simulink model "mCounterWithReset"  (R2021b)
settings: Solver=FixedStepDiscrete  StartTime=0.0  StopTime=10.0  RelTol=1e-3
PreLoadFcn:
  | A=1;
  | 
  | % -------------------------------------------------------------------
  | %  Generated by MATLAB on 17-Oct-2019 16:20:17
  | %  MATLAB version: 9.8.0.1209737 (R2020a) Prerelease
  | % -------------------------------------------------------------------
  | 
  | 
  | main_bus = Simulink.Bus;
  | main_bus.Description = '';
  | main_bus.DataScope = 'Auto';
  | main_bus.HeaderFile = '';
  | main_bus.Alignment = -1;
  | saveVarsTmp{1} = Simulink.BusElement;
  | saveVarsTmp{1}.Name = 'Counter';
  | saveVarsTmp{1}.Complexity = 'real';
  | saveVarsTmp{1}.Dimensions = 1;
  | saveVarsTmp{1}.DataType = 'double';
  | saveVarsTmp{1}.Min = [];
  | saveVarsTmp{1}.Max = [];
  | saveVarsTmp{1}.DimensionsMode = 'Fixed';
  | saveVarsTmp{1}.SamplingMode = 'Sample based';
  | saveVarsTmp{1}.SampleTime = -1;
  | saveVarsTmp{1}.DocUnits = '';
  | saveVarsTmp{1}.Description = '';
  | saveVarsTmp{1}(2, 1) = Simulink.BusElement;
  | saveVarsTmp{1}(2, 1).Name = 'Reset';
  | saveVarsTmp{1}(2, 1).Complexity = 'real';
  | saveVarsTmp{1}(2, 1).Dimensions = 1;
  | saveVarsTmp{1}(2, 1).DataType = 'boolean';
  | saveVarsTmp{1}(2, 1).Min = [];
  | saveVarsTmp{1}(2, 1).Max = [];
  | saveVarsTmp{1}(2, 1).DimensionsMode = 'Fixed';
  | saveVarsTmp{1}(2, 1).SamplingMode = 'Sample based';
  | saveVarsTmp{1}(2, 1).SampleTime = -1;
  | saveVarsTmp{1}(2, 1).DocUnits = '';
  | saveVarsTmp{1}(2, 1).Description = '';
  | main_bus.Elements = saveVarsTmp{1};
  | clear saveVarsTmp;
CloseFcn:
  | clear A main_bus;
settings Model: Creator=nrangava  LastModifiedBy=nrangava
settings SolverCC: AlgebraicLoopSolver=TrustRegion  MaxZcPerStep=1
settings DataIOCC: SaveFormat=StructureWithTime  SaveState=on  DSMLogging=off  OutputSaveName=yout1
settings OptimizationCC: DefaultParameterBehavior=Inlined  EnhancedBackFolding=on  PassReuseOutputArgsAs=Individual arguments  ZeroExternalMemoryAtStartup=off  ZeroInternalMemoryAtStartup=off  OptimizeBlockOrder=speed  DifferentSizesBufferReuse=on  OptimizationCustomize=off  EfficientTunableParamExpr=on
settings DebuggingCC: ParameterTunabilityLossMsg=error  SFMachineParentedDataDiag=warning
settings HardwareCC: TargetBitPerPointer=64  TargetBitPerSizeT=64  TargetBitPerPtrDiffT=64  TargetLongLongMode=on  TargetIntDivRoundTo=Zero  TargetEndianess=LittleEndian  TargetWordSize=64  TargetHWDeviceType=Custom Processor->MATLAB Host Computer  ProdEqTarget=off
settings ModelReferenceCC: UpdateModelReferenceTargets=IfOutOfDate
settings SFSimCC: MATLABDynamicMemAlloc=off
settings RTWCC: Description=Embedded Coder  SystemTargetFile=ert.tlc  TemplateMakefile=ert_default_tmf  RTWVerbose=off  RetainRTWFile=on  TLCAssert=on
settings CodeAppCC: ForceParamTrailComments=on  IgnoreCustomStorageClasses=off  MaxIdLength=64  OperatorAnnotations=on  SimulinkDataObjDesc=on  SFDataObjDesc=on  InsertBlockDesc=on
settings ERTTargetCC: TargetLangStandard=C99 (ISO)  GenerateSampleERTMain=on  CombineOutputUpdateFcns=off  LogVarNameModifier=none  MatFileLogging=on  InlinedParameterPlacement=NonHierarchical  ERTCustomFileTemplate=example_file_process.tlc

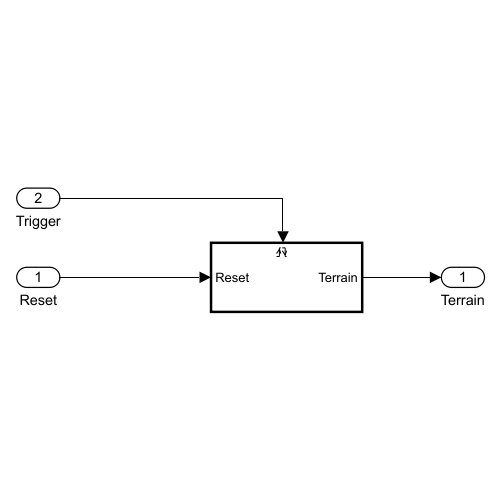
[thumbnail: Simulink's stored preview of the top-level diagram]
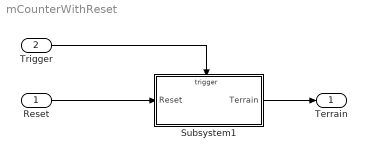
== system mCounterWithReset ==
  Reset : Inport  OutDataTypeStr=boolean
  Trigger : Inport  Port=2  OutDataTypeStr=boolean
  Subsystem1 : Subsystem  TreatAsAtomicUnit=on  VariantControl=A==2
  Terrain : Outport
  wires:
  Reset/1 -> Subsystem1/1(Reset)
  Subsystem1/1(Terrain) -> Terrain/1
  Trigger/1 -> Subsystem1/Trigger

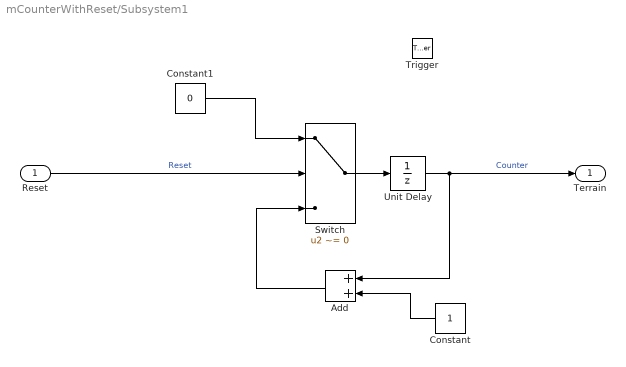
== system mCounterWithReset/Subsystem1 ==
  Reset : Inport
  Trigger : TriggerPort  TriggerType=either  VariantControl=Variant  PortDimensions=1
  Add : Sum
  Constant : Constant
  Constant1 : Constant  Value=0
  Switch : Switch  Criteria=u2 ~= 0
  Unit Delay : UnitDelay  SampleTime=-1  HasFrameUpgradeWarning=on
  Terrain : Outport
  wires:
  Switch/1 -> Unit Delay/1
  Constant1/1 -> Switch/1
  Unit Delay/1 -> Terrain/1, Add/1  "Counter"
  Constant/1 -> Add/2
  Add/1 -> Switch/3
  Reset/1 -> Switch/2  "Reset"
